simulink model "Simscape_Assem"  (R2025a)
settings: Solver=FixedStepAuto  StartTime=0.0  StopTime=7  FixedStep=0.00005  RelTol=1e-3
model workspace: external: MATLAB File C:\Users\ACER\Documents\GitHub\StudioYear2_G13\Studio\Matlab\Simscape\2 model _ with cast rod\Simscape_Assem_DataFile.m (data not in the file)
undefined symbols (not defined in the file or in its folder): smiData, X, Y, Z
libraries: sm_lib x15, nesl_utility x6
settings Model: Creator=ACER  LastModifiedBy=ACER

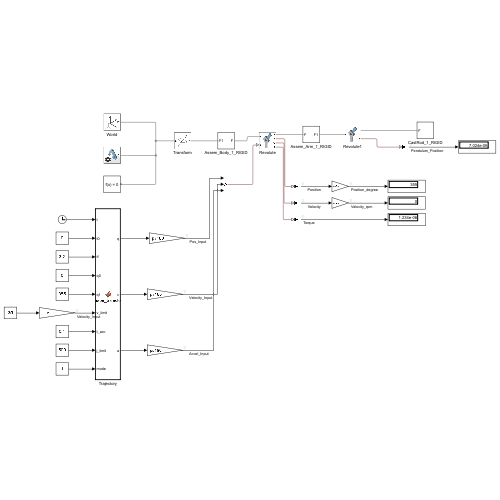
[thumbnail: Simulink's stored preview of the top-level diagram]
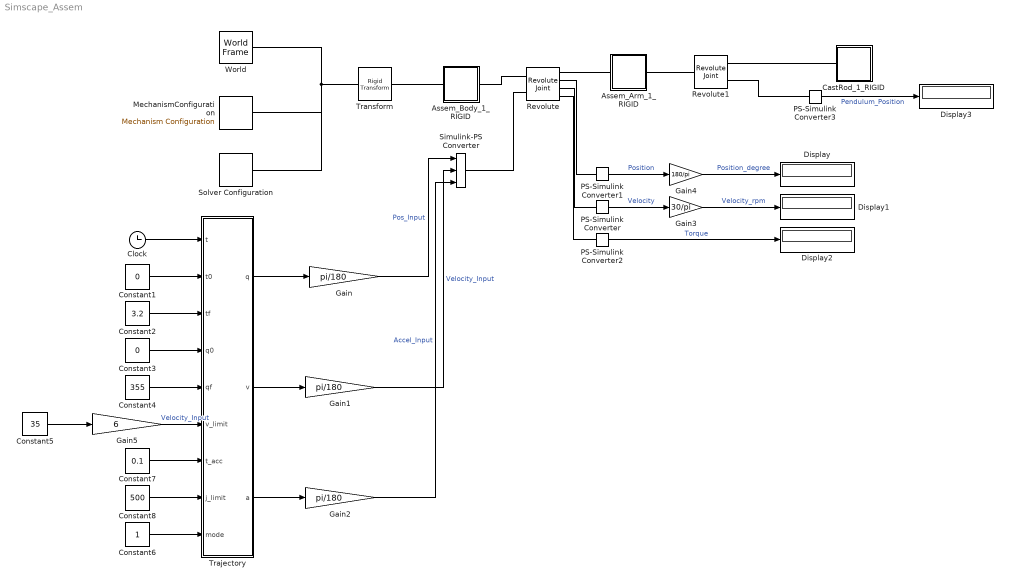
== system Simscape_Assem ==
  Assem_Arm_1_RIGID : Subsystem
  Assem_Body_1_RIGID : Subsystem
  CastRod_1_RIGID : Subsystem
  Clock : Clock
  Constant1 : Constant  Value=0
  Constant2 : Constant  Value=3.2
  Constant3 : Constant  Value=0
  Constant4 : Constant  Value=355
  Constant5 : Constant  Value=35
  Constant6 : Constant
  Constant7 : Constant  Value=0.1
  Constant8 : Constant  Value=500
  Display{,1..3} (4 alike) : Display
  Gain : Gain  Gain=pi/180
  Gain1 : Gain  Gain=pi/180
  Gain2 : Gain  Gain=pi/180
  Gain3 : Gain  Gain=30/pi
  Gain4 : Gain  Gain=180/pi
  Gain5 : Gain  Gain=6
  MechanismConfiguration : sm_lib/Utilities/Mechanism Configuration  UniformGravity=Constant  GravityVector=[0 -9.80665 0]  GravityVectorUnits=m/s^2  LinearizationDelta=0.001  JointModeTransitionNonlinearIterations=2
  PS-Simulink Converter{,1..3} (4 alike) : nesl_utility/PS-Simulink Converter  PhysicalDomain=network_engine_domain  SubClassName=ps_output  LeftPortType=input  RightPortType=output  PseudoPeriodic=off  Frequencies=[]  VectorFormat=inherit  Unit=inherit  AffineConversion=off
  Revolute : sm_lib/Joints/Revolute Joint  JointMode=Normal  CompositeWrenchDir=FollowerOnBase  CompositeWrenchFrame=BaseFrame  SenseConstraintForce=off  SenseConstraintTorque=off  SenseTotalForce=off  SenseTotalTorque=off  PositionTargetSpecify=on  PositionTargetPriority=High  PositionTargetValue=smiData.RevoluteJoint(1).Rz.Pos  PositionTargetValueUnits=deg  VelocityTargetSpecify=off  VelocityTargetPriority=High  VelocityTargetValue=0  VelocityTargetValueUnits=deg/s  EquilibriumPosition=0  EquilibriumPositionUnits=deg  SpringStiffness=0  SpringStiffnessUnits=N*m/deg  DampingCoefficient=0.0021467  DampingCoefficientUnits=N*m/(deg/s)  LowerLimitSpecify=off  LowerLimitBound=-90  LowerLimitBoundUnits=deg  LowerLimitStiffness=1e4  LowerLimitStiffnessUnits=N*m/deg  LowerLimitDamping=10  LowerLimitDampingUnits=N*m/(deg/s)  LowerLimitTransitionRegionWidth=0.1  LowerLimitTransitionRegionWidthUnits=deg  UpperLimitSpecify=off  UpperLimitBound=90  UpperLimitBoundUnits=deg  UpperLimitStiffness=1e4  UpperLimitStiffnessUnits=N*m/deg  UpperLimitDamping=10  UpperLimitDampingUnits=N*m/(deg/s)  UpperLimitTransitionRegionWidth=0.1  UpperLimitTransitionRegionWidthUnits=deg  TorqueActuationMode=ComputedTorque  MotionActuationMode=InputMotion  SensePosition=on  SenseVelocity=on  SenseAcceleration=off  SenseTorqueForce=on  SenseLowerLimitTorqueForce=off  SenseUpperLimitTorqueForce=off
  Revolute1 : sm_lib/Joints/Revolute Joint  JointMode=Normal  CompositeWrenchDir=FollowerOnBase  CompositeWrenchFrame=BaseFrame  SenseConstraintForce=off  SenseConstraintTorque=off  SenseTotalForce=off  SenseTotalTorque=off  PositionTargetSpecify=on  PositionTargetPriority=Low  PositionTargetValue=smiData.RevoluteJoint(2).Rz.Pos  PositionTargetValueUnits=deg  VelocityTargetSpecify=off  VelocityTargetPriority=High  VelocityTargetValue=0  VelocityTargetValueUnits=deg/s  EquilibriumPosition=0  EquilibriumPositionUnits=deg  SpringStiffness=0  SpringStiffnessUnits=N*m/deg  DampingCoefficient=0.0005  DampingCoefficientUnits=N*m/(deg/s)  LowerLimitSpecify=off  LowerLimitBound=-90  LowerLimitBoundUnits=deg  LowerLimitStiffness=1e4  LowerLimitStiffnessUnits=N*m/deg  LowerLimitDamping=10  LowerLimitDampingUnits=N*m/(deg/s)  LowerLimitTransitionRegionWidth=0.1  LowerLimitTransitionRegionWidthUnits=deg  UpperLimitSpecify=off  UpperLimitBound=90  UpperLimitBoundUnits=deg  UpperLimitStiffness=1e4  UpperLimitStiffnessUnits=N*m/deg  UpperLimitDamping=10  UpperLimitDampingUnits=N*m/(deg/s)  UpperLimitTransitionRegionWidth=0.1  UpperLimitTransitionRegionWidthUnits=deg  TorqueActuationMode=NoTorque  MotionActuationMode=ComputedMotion  SensePosition=on  SenseVelocity=off  SenseAcceleration=off  SenseTorqueForce=off  SenseLowerLimitTorqueForce=off  SenseUpperLimitTorqueForce=off
  Simulink-PS Converter : nesl_utility/Simulink-PS Converter  PhysicalDomain=network_engine_domain  SubClassName=ps_input  LeftPortType=input  RightPortType=output  PseudoPeriodic=off  Frequencies=[]  NoiseDistribution=none  NoiseParameters=[]  Unit=1  AffineConversion=off  FilteringAndDerivatives=provide  SimscapeFilterOrder=1  InputFilterTimeConstant=0.001  UdotUserProvided=2
  Solver Configuration : nesl_utility/Solver Configuration  PhysicalDomain=network_engine_domain  SubClassName=solver  LeftPortType=input  RightPortType=generic  Tones=[]  Harmonics=[]  SimulateNoise=off  Profile=off  UseLocalSampling=off  EnableSwitchedLinearOptims=on  FrequencyDomain=off  UseCCode=off  RelTol=0.001  AbsTol=0.001  MinStep=1e-09  ToWorkspace=off  RevertToSquareIcSolve=off  NumHomotopyIterations=100  PhasorMode=off  PhasorModeNumHarmonics=1  ConsistencySolver=NEWTON_XTOL_AFTER_FTOL  IndexReductionMethod=DerivativeReplacement  DoDC=off  ResidualTolerance=1e-09  ConsistencyTolSource=GLOBAL  ConsistencyAbsTol=0.001  ConsistencyRelTol=0.001  ConsistencyTolFactor=0.001  UseLocalSolver=off  LocalSolverChoice=NE_BACKWARD_EULER_ADVANCER  ResolveIndetEquations=on  FunctionEvalNumThread=1  LocalSolverSampleTime=0.001  DoFixedCost=off  MaxNonlinIter=3  MaxModeIter=2  ComputeImpulses=off  ImpulseIterations=2  LinearAlgebra=auto  LinearAlgebraNumThread=0  EquationFormulation=NE_TIME_EF  DelaysMemoryBudget=1024  AutomaticFiltering=on  FilteringTimeConstant=0.001  PartitionStorageMethod=AS_NEEDED  PartitionMemoryBudget=1024  PartitionMethod=ROBUST  MultibodyUseLocalSolver=off  MultibodyLocalSolverChoice=ODE1  MultibodyLocalSolverSampleTime=0.001
  Trajectory : MATLAB Function  TreatAsAtomicUnit=on
  Transform : sm_lib/Frames and Transforms/Rigid Transform  RotationMethod=ArbitraryAxis  FollAlignAxisA=+X  BaseAlignAxisA=+Y  FollAlignAxisB=+Y  BaseAlignAxisB=+Z  RotationStandardAxis=+Z  RotationAngle=smiData.RigidTransform(5).angle  RotationAngleUnits=rad  RotationArbitraryAxis=smiData.RigidTransform(5).axis  RotationSequenceAxes=FollowerAxes  RotationSequence=XYX  RotationSequenceAngles=[0 0 0]  RotationSequenceAnglesUnits=deg  RotationMatrix=[1 0 0;0 1 0;0 0 1]  Quaternion=[1 0 0 0]  TranslationMethod=Cartesian  TranslationCartesianOffset=smiData.RigidTransform(5).translation  TranslationCartesianOffsetUnits=mm  TranslationStandardAxis=+Z  TranslationStandardOffset=0  TranslationStandardOffsetUnits=m  TranslationROffset=0  TranslationROffsetUnits=m  TranslationThetaOffset=0  TranslationThetaOffsetUnits=deg  TranslationZOffset=0  TranslationZOffsetUnits=m
  World : sm_lib/Frames and Transforms/World Frame
  wires:
  Constant1/1 -> Trajectory/2(t0)
  Constant3/1 -> Trajectory/4(q0)
  Constant4/1 -> Trajectory/5(qf)
  Clock/1 -> Trajectory/1(t)
  Constant2/1 -> Trajectory/3(tf)
  Trajectory/1(q) -> Gain/1
  PS-Simulink Converter1/1 -> Gain4/1  "Position"
  PS-Simulink Converter/1 -> Gain3/1  "Velocity"
  Trajectory/2(v) -> Gain1/1
  Trajectory/3(a) -> Gain2/1
  PS-Simulink Converter2/1 -> Display2/1  "Torque"
  PS-Simulink Converter3/1 -> Display3/1  "Pendulum_Position"
  Gain/1 -> Simulink-PS Converter/1  "Pos_Input"
  Gain1/1 -> Simulink-PS Converter/2  "Velocity_Input"
  Gain2/1 -> Simulink-PS Converter/3  "Accel_Input"
  Constant5/1 -> Gain5/1
  Constant6/1 -> Trajectory/9(mode)
  Gain3/1 -> Display1/1  "Velocity_rpm"
  Gain4/1 -> Display/1  "Position_degree"
  Constant7/1 -> Trajectory/7(t_acc)
  Constant8/1 -> Trajectory/8(j_limit)
  Gain5/1 -> Trajectory/6(v_limit)  "Velocity_Input"
  connections:
  Solver Configuration/RConn1 -- MechanismConfiguration/RConn1 -- Transform/LConn1 -- World/RConn1
  Assem_Body_1_RIGID/RConn1 -- Revolute/LConn1
  Assem_Arm_1_RIGID/LConn1 -- Revolute/RConn1
  Assem_Arm_1_RIGID/RConn1 -- Revolute1/LConn1
  CastRod_1_RIGID/LConn1 -- Revolute1/RConn1
  Assem_Body_1_RIGID/LConn1 -- Transform/RConn1
  Simulink-PS Converter/RConn1 -- Revolute/LConn2
  Revolute/RConn2 -- PS-Simulink Converter1/LConn1
  Revolute/RConn3 -- PS-Simulink Converter/LConn1
  Revolute/RConn4 -- PS-Simulink Converter2/LConn1
  PS-Simulink Converter3/LConn1 -- Revolute1/RConn2

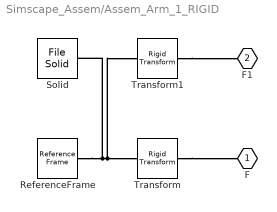
== system Simscape_Assem/Assem_Arm_1_RIGID ==
  ReferenceFrame : sm_lib/Frames and Transforms/Reference Frame
  Solid : sm_lib/Body Elements/File Solid  ExtGeomFileName=Assem_Arm_Default_sldprt.STEP  UnitType=FromFile  ExtGeomFileUnits=m  StepReaderType=HEX  ExportConvexHullGeometry=off  InertiaType=Custom  BasedOnType=DensityFromFile  Density=1000  DensityUnits=kg/m^3  Mass=1  MassUnits=kg  CenterOfMass=[0 0 0]  CenterOfMassUnits=mm  MomentsOfInertia="[0.01  0.5  0.01]"  MomentsOfInertiaUnits=kg*m^2  ProductsOfInertia=[0 0 0]  ProductsOfInertiaUnits=kg*m^2  GraphicType=FromGeometry  MarkerShape=Sphere  MarkerSize=10  GraphicVisPropType=SimpleVisualProperties  GraphicDiffuseColor=smiData.Solid(1).color  GraphicOpacity=smiData.Solid(1).opacity  GraphicSpecularColor=[0.5 0.5 0.5 1.0]  GraphicAmbientColor=[0.15 0.15 0.15 1.0]  GraphicEmissiveColor=[0.0 0.0 0.0 1.0]  GraphicShininess=75  DoExposeReferenceFrame=on  SerializedFrames=<Frames/>
  Transform : sm_lib/Frames and Transforms/Rigid Transform  RotationMethod=ArbitraryAxis  FollAlignAxisA=+X  BaseAlignAxisA=+Y  FollAlignAxisB=+Y  BaseAlignAxisB=+Z  RotationStandardAxis=+Z  RotationAngle=smiData.RigidTransform(2).angle  RotationAngleUnits=rad  RotationArbitraryAxis=smiData.RigidTransform(2).axis  RotationSequenceAxes=FollowerAxes  RotationSequence=XYX  RotationSequenceAngles=[0 0 0]  RotationSequenceAnglesUnits=deg  RotationMatrix=[1 0 0;0 1 0;0 0 1]  Quaternion=[1 0 0 0]  TranslationMethod=Cartesian  TranslationCartesianOffset=smiData.RigidTransform(2).translation  TranslationCartesianOffsetUnits=mm  TranslationStandardAxis=+Z  TranslationStandardOffset=0  TranslationStandardOffsetUnits=m  TranslationROffset=0  TranslationROffsetUnits=m  TranslationThetaOffset=0  TranslationThetaOffsetUnits=deg  TranslationZOffset=0  TranslationZOffsetUnits=m
  Transform1 : sm_lib/Frames and Transforms/Rigid Transform  RotationMethod=ArbitraryAxis  FollAlignAxisA=+X  BaseAlignAxisA=+Y  FollAlignAxisB=+Y  BaseAlignAxisB=+Z  RotationStandardAxis=+Z  RotationAngle=smiData.RigidTransform(3).angle  RotationAngleUnits=rad  RotationArbitraryAxis=smiData.RigidTransform(3).axis  RotationSequenceAxes=FollowerAxes  RotationSequence=XYX  RotationSequenceAngles=[0 0 0]  RotationSequenceAnglesUnits=deg  RotationMatrix=[1 0 0;0 1 0;0 0 1]  Quaternion=[1 0 0 0]  TranslationMethod=Cartesian  TranslationCartesianOffset=smiData.RigidTransform(3).translation  TranslationCartesianOffsetUnits=mm  TranslationStandardAxis=+Z  TranslationStandardOffset=0  TranslationStandardOffsetUnits=m  TranslationROffset=0  TranslationROffsetUnits=m  TranslationThetaOffset=0  TranslationThetaOffsetUnits=deg  TranslationZOffset=0  TranslationZOffsetUnits=m
  F : PMIOPort  Side=Left
  F1 : PMIOPort  Port=2  Side=Right
  connections:
  Solid/RConn1 -- ReferenceFrame/RConn1 -- Transform/LConn1 -- Transform1/LConn1
  Transform/RConn1 -- F/RConn1
  Transform1/RConn1 -- F1/RConn1

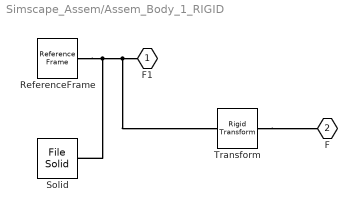
== system Simscape_Assem/Assem_Body_1_RIGID ==
  ReferenceFrame : sm_lib/Frames and Transforms/Reference Frame
  Solid : sm_lib/Body Elements/File Solid  ExtGeomFileName=Assem_Body_Default_sldprt.STEP  UnitType=FromFile  ExtGeomFileUnits=m  StepReaderType=HEX  ExportConvexHullGeometry=off  InertiaType=Custom  BasedOnType=DensityFromFile  Density=1000  DensityUnits=kg/m^3  Mass=smiData.Solid(2).mass  MassUnits=kg  CenterOfMass=smiData.Solid(2).CoM  CenterOfMassUnits=mm  MomentsOfInertia=smiData.Solid(2).MoI  MomentsOfInertiaUnits=kg*mm^2  ProductsOfInertia=smiData.Solid(2).PoI  ProductsOfInertiaUnits=kg*mm^2  GraphicType=FromGeometry  MarkerShape=Sphere  MarkerSize=10  GraphicVisPropType=SimpleVisualProperties  GraphicDiffuseColor=smiData.Solid(2).color  GraphicOpacity=smiData.Solid(2).opacity  GraphicSpecularColor=[0.5 0.5 0.5 1.0]  GraphicAmbientColor=[0.15 0.15 0.15 1.0]  GraphicEmissiveColor=[0.0 0.0 0.0 1.0]  GraphicShininess=75  DoExposeReferenceFrame=on  SerializedFrames=<Frames/>
  Transform : sm_lib/Frames and Transforms/Rigid Transform  RotationMethod=ArbitraryAxis  FollAlignAxisA=+X  BaseAlignAxisA=+Y  FollAlignAxisB=+Y  BaseAlignAxisB=+Z  RotationStandardAxis=+Z  RotationAngle=smiData.RigidTransform(1).angle  RotationAngleUnits=rad  RotationArbitraryAxis=smiData.RigidTransform(1).axis  RotationSequenceAxes=FollowerAxes  RotationSequence=XYX  RotationSequenceAngles=[0 0 0]  RotationSequenceAnglesUnits=deg  RotationMatrix=[1 0 0;0 1 0;0 0 1]  Quaternion=[1 0 0 0]  TranslationMethod=Cartesian  TranslationCartesianOffset=smiData.RigidTransform(1).translation  TranslationCartesianOffsetUnits=mm  TranslationStandardAxis=+Z  TranslationStandardOffset=0  TranslationStandardOffsetUnits=m  TranslationROffset=0  TranslationROffsetUnits=m  TranslationThetaOffset=0  TranslationThetaOffsetUnits=deg  TranslationZOffset=0  TranslationZOffsetUnits=m
  F1 : PMIOPort  Side=Left
  F : PMIOPort  Port=2  Side=Right
  connections:
  Solid/RConn1 -- ReferenceFrame/RConn1 -- Transform/LConn1 -- F1/RConn1
  Transform/RConn1 -- F/RConn1

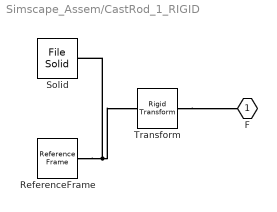
== system Simscape_Assem/CastRod_1_RIGID ==
  ReferenceFrame : sm_lib/Frames and Transforms/Reference Frame
  Solid : sm_lib/Body Elements/File Solid  ExtGeomFileName=CastRod_Default_sldprt.STEP  UnitType=FromFile  ExtGeomFileUnits=m  StepReaderType=HEX  ExportConvexHullGeometry=off  InertiaType=Custom  BasedOnType=DensityFromFile  Density=1000  DensityUnits=kg/m^3  Mass=smiData.Solid(3).mass  MassUnits=kg  CenterOfMass=smiData.Solid(3).CoM  CenterOfMassUnits=mm  MomentsOfInertia=smiData.Solid(3).MoI  MomentsOfInertiaUnits=kg*mm^2  ProductsOfInertia=smiData.Solid(3).PoI  ProductsOfInertiaUnits=kg*mm^2  GraphicType=FromGeometry  MarkerShape=Sphere  MarkerSize=10  GraphicVisPropType=SimpleVisualProperties  GraphicDiffuseColor=smiData.Solid(3).color  GraphicOpacity=smiData.Solid(3).opacity  GraphicSpecularColor=[0.5 0.5 0.5 1.0]  GraphicAmbientColor=[0.15 0.15 0.15 1.0]  GraphicEmissiveColor=[0.0 0.0 0.0 1.0]  GraphicShininess=75  DoExposeReferenceFrame=on  SerializedFrames=<Frames/>
  Transform : sm_lib/Frames and Transforms/Rigid Transform  RotationMethod=ArbitraryAxis  FollAlignAxisA=+X  BaseAlignAxisA=+Y  FollAlignAxisB=+Y  BaseAlignAxisB=+Z  RotationStandardAxis=+Z  RotationAngle=smiData.RigidTransform(4).angle  RotationAngleUnits=rad  RotationArbitraryAxis=smiData.RigidTransform(4).axis  RotationSequenceAxes=FollowerAxes  RotationSequence=XYX  RotationSequenceAngles=[0 0 0]  RotationSequenceAnglesUnits=deg  RotationMatrix=[1 0 0;0 1 0;0 0 1]  Quaternion=[1 0 0 0]  TranslationMethod=Cartesian  TranslationCartesianOffset=smiData.RigidTransform(4).translation  TranslationCartesianOffsetUnits=mm  TranslationStandardAxis=+Z  TranslationStandardOffset=0  TranslationStandardOffsetUnits=m  TranslationROffset=0  TranslationROffsetUnits=m  TranslationThetaOffset=0  TranslationThetaOffsetUnits=deg  TranslationZOffset=0  TranslationZOffsetUnits=m
  F : PMIOPort  Side=Left
  connections:
  Solid/RConn1 -- ReferenceFrame/RConn1 -- Transform/LConn1
  Transform/RConn1 -- F/RConn1

== matlab function Simscape_Assem/Trajectory ==
  data: t input; q output; t0 input; tf input; q0 input; qf input; v output; a output; v_limit input; t_acc input; j_limit input; mode input
function [q, v, a] = master_trajectory(t, t0, tf, q0, qf, v_limit, t_acc, j_limit, mode)
    % Inputs:
    % t       - Current simulation time
    % t0      - Start time of the motion
    % tf      - End time (Ignored in Mode 3)
    % q0      - Starting position 
    % qf      - Final position
    % v_limit - Maximum velocity (Used in Mode 3)
    % t_acc   - Desired Acceleration Time (Used in Mode 3)
    % j_limit - Maximum jerk / Accel ramp rate (Used in Mode 3)
    % mode    - 1: 5th-Order Poly, 2: 7th-Order Poly, 3: Time-Optimal S-Curve (Auto-Accel)
    
    % Initialize outputs safely
    q = q0;
    v = 0;
    a = 0;
    
    % Before start time
    if t <= t0
        return;
    end
    
    % Shared Variables
    tau = t - t0;
    dq = qf - q0;
    D = abs(dq);
    dir = sign(dq);
    if dir == 0
        dir = 1; % Safety fallback
    end
    
    % ===========================================
    % MODE 1: 5th-Order Polynomial (Fixed Time)
    % ===========================================
    if mode == 1
        T = tf - t0;
        if T <= 0 || tau >= T
            q = qf;
        else
            u = tau / T;
            q = q0 + dq * (10*u^3 - 15*u^4 + 6*u^5);
            v = (dq / T) * (30*u^2 - 60*u^3 + 30*u^4);
            a = (dq / T^2) * (60*u - 180*u^2 + 120*u^3);
        end
        
    % ===========================================
    % MODE 2: 7th-Order Polynomial (Fixed Time)
    % ===========================================
    elseif mode == 2
        T = tf - t0;
        if T <= 0 || tau >= T
            q = qf;
        else
            u = tau / T;
            
            s = -20*u^7 + 70*u^6 - 84*u^5 + 35*u^4;
            q = q0 + dq * s;
            
            ds = -140*u^6 + 420*u^5 - 420*u^4 + 140*u^3;
            v = (dq / T) * ds;
            
            dds = -840*u^5 + 2100*u^4 - 1680*u^3 + 420*u^2;
            a = (dq / T^2) * dds;
        end
        
    % ===========================================
    % MODE 3: Auto-Accel S-Curve (Fast as possible)
    % ===========================================
    elseif mode == 3
        Vmax = abs(v_limit);
        Tacc = abs(t_acc); 
        Jmax = abs(j_limit);
        
        % Safety check
        if Vmax == 0 || Jmax == 0 || Tacc == 0 || D == 0
            q = q0;
        else
            % 1. Automatically find Amax based on Tacc
            % Minimum possible time to reach Vmax without constant accel phase
            Tacc_min = 2 * sqrt(Vmax / Jmax);
            
            % Clamp user input if impossible
            if Tacc < Tacc_min
                Tacc = Tacc_min;
            end
            
            % Solve for tj (jerk time)
            tj = (Tacc - sqrt(Tacc^2 - 4 * (Vmax / Jmax))) / 2;
            
            % THE AUTOMATICALLY FOUND ACCELERATION LIMIT
            Amax = Jmax * tj;
            
            % Full acceleration phase time
            ta_full = Tacc - 2*tj;
            
            % Distance required just to accelerate
            d_acc = Vmax * (tj + ta_full / 2);
            
            % 2. Check if target is far enough to reach max velocity
            if D >= 2 * d_acc
                tv = (D - 2 * d_acc) / Vmax;
                ta = ta_full;
            else
                tv = 0;
                % If we can't reach Vmax, check if we even reach our found Amax
                if D < 2 * Amax^3 / Jmax^2
                    tj = (D / (2 * Jmax))^(1/3);
                    ta = 0;
                    Vmax = Jmax * tj^2;
                else
                    tj = Amax / Jmax;
                    b = 3 * tj;
                    c = 2 * tj^2 - D / Amax;
                    ta = (-b + sqrt(b^2 - 4 * c)) / 2;
                    Vmax = Amax * tj + Amax * ta;
                end
            end
            
            % 3. Calculate internal time nodes
            t1 = tj;
            t2 = tj + ta;
            t3 = 2*tj + ta;
            t4 = t3 + tv;
            t5 = t4 + tj;
            t6 = t5 + ta;
            t7 = t6 + tj;
            
            % If the calculated dynamic time has passed
            if tau >= t7
                q = qf;
            else
                % 4. Build Kinematic Sequence based on what was reachable
                A = Jmax * tj; % The peak acceleration actually reached
                
                v1 = 0.5 * Jmax * tj^2;
                q1 = (1/6) * Jmax * tj^3;
                
                v2 = v1 + A * ta;
                q2 = q1 + v1 * ta + 0.5 * A * ta^2;
                
                v3 = Vmax;
                q3 = q2 + v2 * tj + 0.5 * A * tj^2 - (1/6) * Jmax * tj^3;
                
                v4 = Vmax;
                q4 = q3 + Vmax * tv;
                
                v5 = v2;
                q5 = q4 + v4 * tj - (1/6) * Jmax * tj^3;
                
                v6 = v1;
                q6 = q5 + v5 * ta - 0.5 * A * ta^2;
                
                % 5. Execute Piecewise Profiles
                if tau < t1
                    a_mag = Jmax * tau;
                    v_mag = 0.5 * Jmax * tau^2;
                    q_mag = (1/6) * Jmax * tau^3;
                elseif tau < t2
                    dt = tau - t1;
                    a_mag = A;
                    v_mag = v1 + A * dt;
                    q_mag = q1 + v1 * dt + 0.5 * A * dt^2;
                elseif tau < t3
                    dt = tau - t2;
                    a_mag = A - Jmax * dt;
                    v_mag = v2 + A * dt - 0.5 * Jmax * dt^2;
                    q_mag = q2 + v2 * dt + 0.5 * A * dt^2 - (1/6) * Jmax * dt^3;
                elseif tau < t4
                    dt = tau - t3;
                    a_mag = 0;
                    v_mag = Vmax;
                    q_mag = q3 + Vmax * dt;
                elseif tau < t5
                    dt = tau - t4;
                    a_mag = -Jmax * dt;
                    v_mag = v4 - 0.5 * Jmax * dt^2;
                    q_mag = q4 + v4 * dt - (1/6) * Jmax * dt^3;
                elseif tau < t6
                    dt = tau - t5;
                    a_mag = -A;
                    v_mag = v5 - A * dt;
                    q_mag = q5 + v5 * dt - 0.5 * A * dt^2;
                else
                    dt = tau - t6;
                    a_mag = -A + Jmax * dt;
                    v_mag = v6 - A * dt + 0.5 * Jmax * dt^2;
                    q_mag = q6 + v6 * dt - 0.5 * A * dt^2 + (1/6) * Jmax * dt^3;
                end
                
                q = q0 + dir * q_mag;
                v = dir * v_mag;
                a = dir * a_mag;
            end
        end
        
    % Default fallback
    else
        q = q0;
    end
end
